simulink model "iface"  (R2018b)
settings: Solver=FixedStepDiscrete  StartTime=0.0  StopTime=10.0  RelTol=1e-3
undefined symbols (not defined in the file): myBool, myBool2, myInteger, myInteger2, myReal, myReal2, mySeqOfVar, mySeqOfVar2
settings Model: Creator=matlab  LastModifiedBy=matlab
settings DataIOCC: SaveOutput=off  SignalLogging=off  SaveTime=off
settings OptimizationCC: DefaultParameterBehavior=Inlined  EnhancedBackFolding=on  PassReuseOutputArgsAs=Individual arguments  OptimizeBlockOrder=speed  DifferentSizesBufferReuse=on  OptimizationCustomize=off
settings DebuggingCC: ParameterTunabilityLossMsg=error
settings SFSimCC: MATLABDynamicMemAlloc=off
settings RTWCC: SystemTargetFile=ert.tlc  TemplateMakefile=ert_default_tmf  PostCodeGenCommand=packNGo(buildInfo);  GenerateReport=on  IncludeHyperlinkInReport=on  LaunchReport=on  GenerateTraceInfo=on  GenerateTraceReport=on  GenerateTraceReportSl=on  GenerateTraceReportSf=on  GenerateTraceReportEml=on
settings CodeAppCC: ForceParamTrailComments=on  IgnoreCustomStorageClasses=off  OperatorAnnotations=on  SimulinkDataObjDesc=on  SFDataObjDesc=on  InsertBlockDesc=on
settings ERTTargetCC: TargetLangStandard=C99 (ISO)  GenerateSampleERTMain=on  InlinedParameterPlacement=NonHierarchical  ERTCustomFileTemplate=example_file_process.tlc

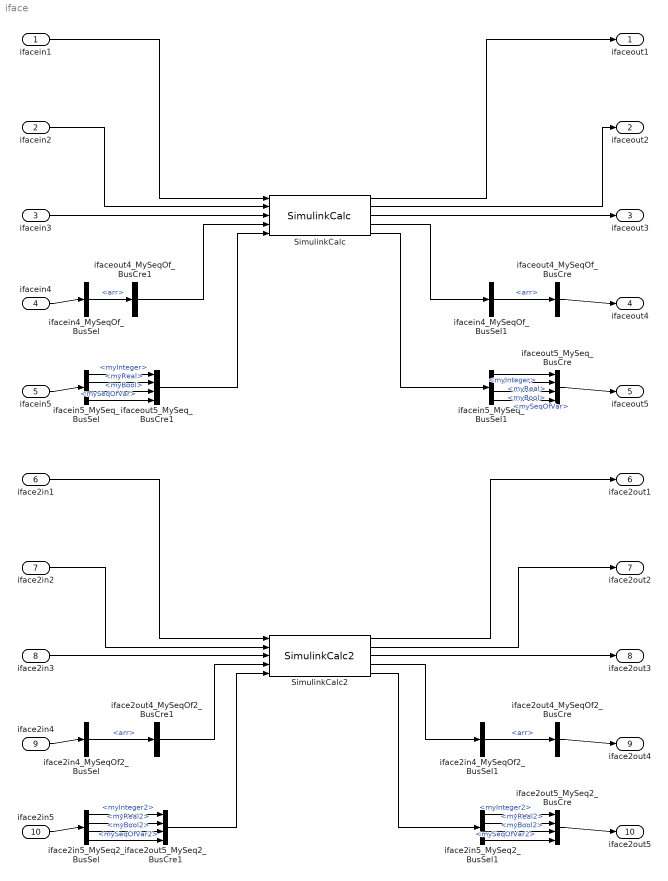
== system iface ==
  ifacein1 : Inport  OutDataTypeStr=MyInteger  BusOutputAsStruct=on
  ifacein2 : Inport  Port=2  OutDataTypeStr=MyReal  BusOutputAsStruct=on
  ifacein3 : Inport  Port=3  OutDataTypeStr=MyBool  BusOutputAsStruct=on
  ifacein4 : Inport  Port=4  OutDataTypeStr=Bus: MySeqOf  BusOutputAsStruct=on
  ifacein5 : Inport  Port=5  OutDataTypeStr=Bus: MySeq  BusOutputAsStruct=on
  iface2in1 : Inport  Port=6  OutDataTypeStr=MyInteger2  BusOutputAsStruct=on
  iface2in2 : Inport  Port=7  OutDataTypeStr=MyReal2  BusOutputAsStruct=on
  iface2in3 : Inport  Port=8  OutDataTypeStr=MyBool2  BusOutputAsStruct=on
  iface2in4 : Inport  Port=9  OutDataTypeStr=Bus: MySeqOf2  BusOutputAsStruct=on
  iface2in5 : Inport  Port=10  OutDataTypeStr=Bus: MySeq2  BusOutputAsStruct=on
  SimulinkCalc : S-Function  FunctionName=SimulinkCalc  SFunctionDeploymentMode=off  EnableBusSupport=off  mask(Legacy Function){SFunctionSpec=void simulink_RI_calc(MyInteger u1[1], MyReal u2[1], MyBool u3[1], MySeqOf u4[1], MySeq u5[1], MyInteger y1[1], MyReal y2[1], MyBool y3[1], MySeqOf y4[1], MySeq y5[1]), ShowSpec=off}
      mask prompts: ShowSpec "Display function specification"
      mask help:
      | This block allows you to call the legacy functions specified by the following Legacy Code Tool definition:
      | def.SFunctionName = 'SimulinkCalc';
      | def.OutputFcnSpec = 'void simulink_RI_calc(MyInteger u1[1], MyReal u2[1], MyBool u3[1], MySeqOf u4[1], MySeq u5[1], MyInteger y1[1], MyReal y2[1], MyBool y3[1], MySeqOf y4[1], MySeq y5[1])';
      | def.HeaderFiles = {'simulink_invoke_ri.h'};
      | def.SourceFiles = {'simulink_invoke_ri.c'};
      | def.IncPaths = {'..\..\..\dataview\C'};
      mask Help: <p>This block was generated automatically by the Legacy Code Tool. For detailed help on this tool, call<a href="matlab:legacy_code('help')"> legacy_code('help')</a>.</p>
      mask Callback ShowSpec:
      | if strcmp(get_param(gcbh, 'ShowSpec'), 'on')
      |   set_param(gcbh, 'MaskDisplay', sprintf('fprintf(''%s'');', get_param(gcbh, 'SFunctionSpec')));
      | else
      |   set_param(gcbh, 'MaskDisplay', sprintf('fprintf(''%s'');', get_param(gcbh, 'FunctionName')));
      | end
      mask Display: fprintf('SimulinkCalc');
  SimulinkCalc2 : S-Function  FunctionName=SimulinkCalc2  SFunctionDeploymentMode=off  EnableBusSupport=off  mask(Legacy Function){SFunctionSpec=void simulink_RI_calc2(MyInteger2 u1[1], MyReal2 u2[1], MyBool2 u3[1], MySeqOf2 u4[1], MySeq2 u5[1], MyInteger2 y1[1], MyReal2 y2[1], MyBool2 y3[1], MySeqOf2 y4[1], MySeq2 y5[1]), ShowSpec=off}
      mask prompts: ShowSpec "Display function specification"
      mask help:
      | This block allows you to call the legacy functions specified by the following Legacy Code Tool definition:
      | def.SFunctionName = 'SimulinkCalc2';
      | def.OutputFcnSpec = 'void simulink_RI_calc2(MyInteger2 u1[1], MyReal2 u2[1], MyBool2 u3[1], MySeqOf2 u4[1], MySeq2 u5[1], MyInteger2 y1[1], MyReal2 y2[1], MyBool2 y3[1], MySeqOf2 y4[1], MySeq2 y5[1])';
      | def.HeaderFiles = {'simulink_invoke_ri.h'};
      | def.SourceFiles = {'simulink_invoke_ri.c'};
      | def.IncPaths = {'..\..\..\dataview\C'};
      mask Help: <p>This block was generated automatically by the Legacy Code Tool. For detailed help on this tool, call<a href="matlab:legacy_code('help')"> legacy_code('help')</a>.</p>
      mask Callback ShowSpec:
      | if strcmp(get_param(gcbh, 'ShowSpec'), 'on')
      |   set_param(gcbh, 'MaskDisplay', sprintf('fprintf(''%s'');', get_param(gcbh, 'SFunctionSpec')));
      | else
      |   set_param(gcbh, 'MaskDisplay', sprintf('fprintf(''%s'');', get_param(gcbh, 'FunctionName')));
      | end
      mask Display: fprintf('SimulinkCalc2');
  iface2in4_MySeqOf2_BusSel : BusSelector  OutputSignals=arr
  iface2in4_MySeqOf2_BusSel1 : BusSelector  OutputSignals=arr
  iface2in5_MySeq2_BusSel : BusSelector  OutputSignals=myInteger2,myReal2,myBool2,mySeqOfVar2
  iface2in5_MySeq2_BusSel1 : BusSelector  OutputSignals=myInteger2,myReal2,myBool2,mySeqOfVar2
  iface2out4_MySeqOf2_BusCre : BusCreator  Inputs=1  OutDataTypeStr=Bus: MySeqOf2  NonVirtualBus=on
  iface2out4_MySeqOf2_BusCre1 : BusCreator  Inputs=1  OutDataTypeStr=Bus: MySeqOf2  NonVirtualBus=on
  iface2out5_MySeq2_BusCre : BusCreator  Inputs=myInteger2,myReal2,myBool2,mySeqOfVar2  OutDataTypeStr=Bus: MySeq2  NonVirtualBus=on
  iface2out5_MySeq2_BusCre1 : BusCreator  Inputs=myInteger2,myReal2,myBool2,mySeqOfVar2  OutDataTypeStr=Bus: MySeq2  NonVirtualBus=on
  ifacein4_MySeqOf_BusSel : BusSelector  OutputSignals=arr
  ifacein4_MySeqOf_BusSel1 : BusSelector  OutputSignals=arr
  ifacein5_MySeq_BusSel : BusSelector  OutputSignals=myInteger,myReal,myBool,mySeqOfVar
  ifacein5_MySeq_BusSel1 : BusSelector  OutputSignals=myInteger,myReal,myBool,mySeqOfVar
  ifaceout4_MySeqOf_BusCre : BusCreator  Inputs=1  OutDataTypeStr=Bus: MySeqOf  NonVirtualBus=on
  ifaceout4_MySeqOf_BusCre1 : BusCreator  Inputs=1  OutDataTypeStr=Bus: MySeqOf  NonVirtualBus=on
  ifaceout5_MySeq_BusCre : BusCreator  Inputs=myInteger,myReal,myBool,mySeqOfVar  OutDataTypeStr=Bus: MySeq  NonVirtualBus=on
  ifaceout5_MySeq_BusCre1 : BusCreator  Inputs=myInteger,myReal,myBool,mySeqOfVar  OutDataTypeStr=Bus: MySeq  NonVirtualBus=on
  ifaceout1 : Outport  OutDataTypeStr=MyInteger
  ifaceout2 : Outport  Port=2  OutDataTypeStr=MyReal
  ifaceout3 : Outport  Port=3  OutDataTypeStr=MyBool
  ifaceout4 : Outport  Port=4  OutDataTypeStr=Bus: MySeqOf  BusOutputAsStruct=on
  ifaceout5 : Outport  Port=5  OutDataTypeStr=Bus: MySeq  BusOutputAsStruct=on
  iface2out1 : Outport  Port=6  OutDataTypeStr=MyInteger2
  iface2out2 : Outport  Port=7  OutDataTypeStr=MyReal2
  iface2out3 : Outport  Port=8  OutDataTypeStr=MyBool2
  iface2out4 : Outport  Port=9  OutDataTypeStr=Bus: MySeqOf2  BusOutputAsStruct=on
  iface2out5 : Outport  Port=10  OutDataTypeStr=Bus: MySeq2  BusOutputAsStruct=on
  wires:
  ifacein4/1 -> ifacein4_MySeqOf_BusSel/1
  ifacein5/1 -> ifacein5_MySeq_BusSel/1
  iface2in4/1 -> iface2in4_MySeqOf2_BusSel/1
  iface2in5/1 -> iface2in5_MySeq2_BusSel/1
  ifaceout4_MySeqOf_BusCre/1 -> ifaceout4/1
  ifaceout5_MySeq_BusCre/1 -> ifaceout5/1
  iface2out4_MySeqOf2_BusCre/1 -> iface2out4/1
  iface2out5_MySeq2_BusCre/1 -> iface2out5/1
  ifacein1/1 -> SimulinkCalc/1
  ifacein2/1 -> SimulinkCalc/2
  ifacein3/1 -> SimulinkCalc/3
  SimulinkCalc/3 -> ifaceout3/1
  SimulinkCalc/2 -> ifaceout2/1
  SimulinkCalc/1 -> ifaceout1/1
  ifaceout5_MySeq_BusCre1/1 -> SimulinkCalc/5
  ifaceout4_MySeqOf_BusCre1/1 -> SimulinkCalc/4
  ifacein4_MySeqOf_BusSel/1 -> ifaceout4_MySeqOf_BusCre1/1  "<arr>"
  ifacein5_MySeq_BusSel/1 -> ifaceout5_MySeq_BusCre1/1  "<myInteger>"
  ifacein5_MySeq_BusSel/2 -> ifaceout5_MySeq_BusCre1/2  "<myReal>"
  ifacein5_MySeq_BusSel/3 -> ifaceout5_MySeq_BusCre1/3  "<myBool>"
  ifacein5_MySeq_BusSel/4 -> ifaceout5_MySeq_BusCre1/4  "<mySeqOfVar>"
  ifacein5_MySeq_BusSel1/1 -> ifaceout5_MySeq_BusCre/1  "<myInteger>"
  ifacein4_MySeqOf_BusSel1/1 -> ifaceout4_MySeqOf_BusCre/1  "<arr>"
  ifacein5_MySeq_BusSel1/2 -> ifaceout5_MySeq_BusCre/2  "<myReal>"
  ifacein5_MySeq_BusSel1/4 -> ifaceout5_MySeq_BusCre/4  "<mySeqOfVar>"
  ifacein5_MySeq_BusSel1/3 -> ifaceout5_MySeq_BusCre/3  "<myBool>"
  SimulinkCalc/5 -> ifacein5_MySeq_BusSel1/1
  SimulinkCalc/4 -> ifacein4_MySeqOf_BusSel1/1
  iface2in1/1 -> SimulinkCalc2/1
  iface2in2/1 -> SimulinkCalc2/2
  iface2in3/1 -> SimulinkCalc2/3
  SimulinkCalc2/1 -> iface2out1/1
  SimulinkCalc2/2 -> iface2out2/1
  SimulinkCalc2/3 -> iface2out3/1
  iface2out5_MySeq2_BusCre1/1 -> SimulinkCalc2/5
  iface2out4_MySeqOf2_BusCre1/1 -> SimulinkCalc2/4
  iface2in4_MySeqOf2_BusSel/1 -> iface2out4_MySeqOf2_BusCre1/1  "<arr>"
  iface2in5_MySeq2_BusSel/1 -> iface2out5_MySeq2_BusCre1/1  "<myInteger2>"
  iface2in5_MySeq2_BusSel/2 -> iface2out5_MySeq2_BusCre1/2  "<myReal2>"
  iface2in5_MySeq2_BusSel/3 -> iface2out5_MySeq2_BusCre1/3  "<myBool2>"
  iface2in5_MySeq2_BusSel/4 -> iface2out5_MySeq2_BusCre1/4  "<mySeqOfVar2>"
  iface2in5_MySeq2_BusSel1/2 -> iface2out5_MySeq2_BusCre/2  "<myReal2>"
  iface2in5_MySeq2_BusSel1/3 -> iface2out5_MySeq2_BusCre/3  "<myBool2>"
  SimulinkCalc2/5 -> iface2in5_MySeq2_BusSel1/1
  iface2in5_MySeq2_BusSel1/1 -> iface2out5_MySeq2_BusCre/1  "<myInteger2>"
  iface2in5_MySeq2_BusSel1/4 -> iface2out5_MySeq2_BusCre/4  "<mySeqOfVar2>"
  iface2in4_MySeqOf2_BusSel1/1 -> iface2out4_MySeqOf2_BusCre/1  "<arr>"
  SimulinkCalc2/4 -> iface2in4_MySeqOf2_BusSel1/1
